simulink model "derpage6"  (R2015b)
settings: Solver=FixedStepDiscrete  SolverMode=SingleTasking  StartTime=0.0  StopTime=(12+350)*8  RelTol=1e-3
undefined symbols (not defined in the file or in its folder): rcosine
libraries: dspsrcs4 x2, dspsigops x2, dspstat3 x1
settings Model: Creator=coltmt  LastModifiedBy=coltmt

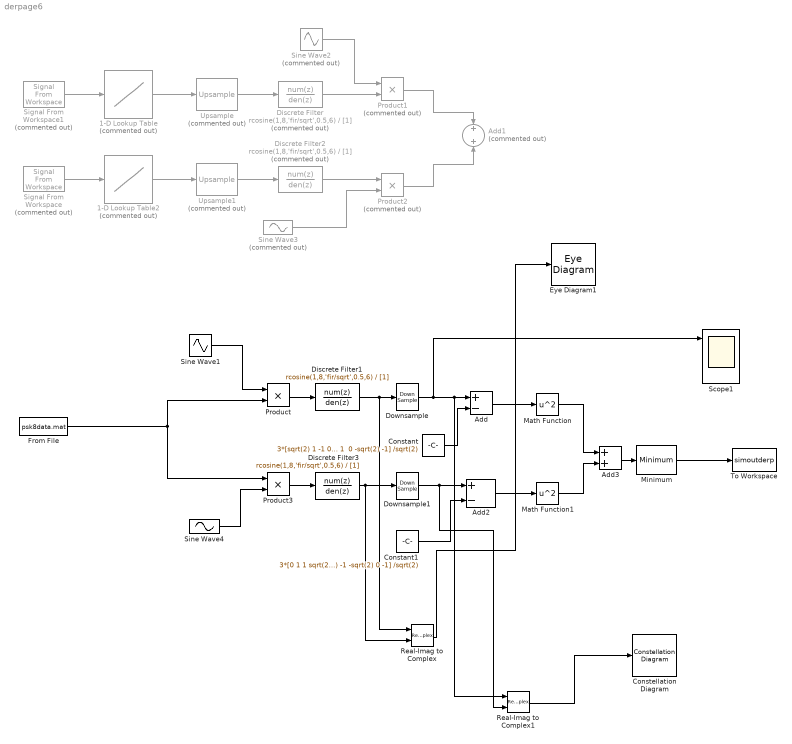
== system derpage6 ==
  1-D Lookup Table : Lookup_n-D  Commented=on  NumberOfTableDimensions=1  BreakpointsForDimension1=[0 1 2 3]  Table=[1 -1 1 -1]*3/sqrt(2)  InternalRulePriority=Speed  RndMeth=Simplest  InputSameDT=on
  1-D Lookup Table2 : Lookup_n-D  Commented=on  NumberOfTableDimensions=1  BreakpointsForDimension1=[0 1 2 3]  Table=[1 1 -1 -1]*3/sqrt(2)  InternalRulePriority=Speed  RndMeth=Simplest  InputSameDT=on
  Add : Sum  Inputs=+-
  Add1 : Sum  Commented=on
  Add2 : Sum  Inputs=+-
  Add3 : Sum
  Constant : Constant  Value="3*[sqrt(2) 1 -1 0 1  0 -sqrt(2) -1] /sqrt(2)"
  Constant1 : Constant  Value=3*[0 1 1 sqrt(2) -1 -sqrt(2) 0 -1] /sqrt(2)
  Constellation Diagram : ConstellationDiagram
  Discrete Filter : DiscreteFilter  Commented=on  Numerator=rcosine(1,8,'fir/sqrt',0.5,6)  Denominator=[1]
  Discrete Filter1 : DiscreteFilter  Numerator=rcosine(1,8,'fir/sqrt',0.5,6)  Denominator=[1]
  Discrete Filter2 : DiscreteFilter  Commented=on  Numerator=rcosine(1,8,'fir/sqrt',0.5,6)  Denominator=[1]
  Discrete Filter3 : DiscreteFilter  Numerator=rcosine(1,8,'fir/sqrt',0.5,6)  Denominator=[1]
  Downsample : DownSample  N=8  InputProcessing=Inherited (this choice will be removed - see release notes)  RateOptions=Allow multirate processing
  Downsample1 : DownSample  N=8  InputProcessing=Inherited (this choice will be removed - see release notes)  RateOptions=Allow multirate processing
  Eye Diagram1 : EyeDiagram
  From File : FromFile  FileName=psk8data.mat  SampleTime=1
  Math Function : Math  Operator=square  SaturateOnIntegerOverflow=on
  Math Function1 : Math  Operator=square  SaturateOnIntegerOverflow=on
  Minimum : dspstat3/Minimum  fcn=Index  reset=None  InputProcessing=Columns as channels (frame based)  indexBase=Zero  operateOver=Each column  Dimension=1  operation=minimum  roiEnable=off  roiType=Rectangles  roiPortion=Entire ROI  roiOutput=Individual statistics for each ROI  roiFlag=off  roundingMode=Floor  overflowMode=off
  Product : Product
  Product1 : Product  Commented=on
  Product2 : Product  Commented=on
  Product3 : Product
  Real-Imag to Complex : RealImagToComplex
  Real-Imag to Complex1 : RealImagToComplex
  Scope1 : Scope  NumInputPorts=3
  Signal From Workspace : dspsrcs4/Signal From Workspace  Commented=on  X=[0 2 1 3]  Ts=8  nsamps=1  OutputAfterFinalValue=Setting to zero  ignoreOrWarnInputAndFrameLengths=off  OutputFrames=off
  Signal From Workspace1 : dspsrcs4/Signal From Workspace  Commented=on  X=[0 2 1 3]  Ts=8  nsamps=1  OutputAfterFinalValue=Setting to zero  ignoreOrWarnInputAndFrameLengths=off  OutputFrames=off
  Sine Wave1 : Sin  Amplitude=sqrt(2)  Frequency=2*pi/4  Phase=pi/2  SampleTime=1
  Sine Wave2 : Sin  Commented=on  Amplitude=sqrt(2)  Frequency=2*pi/4  Phase=pi/2  SampleTime=1
  Sine Wave3 : Sin  Commented=on  Amplitude=-sqrt(2)  Frequency=2*pi/4  SampleTime=1
  Sine Wave4 : Sin  Amplitude=-sqrt(2)  Frequency=2*pi/4  SampleTime=1
  To Workspace : ToWorkspace  VariableName=simoutderp  SampleTime=-1
      settings: Save2DSignal=2-D array (concatenate along first dimension)
  Upsample : dspsigops/Upsample  Commented=on  N=8  phase=0  InputProcessing=Inherited (this choice will be removed - see release notes)  RateOptions=Allow multirate processing  ic=0  mode=Unused parameter value
  Upsample1 : dspsigops/Upsample  Commented=on  N=8  phase=0  InputProcessing=Inherited (this choice will be removed - see release notes)  RateOptions=Allow multirate processing  ic=0  mode=Unused parameter value
  wires:
  Signal From Workspace1/1 -> 1-D Lookup Table/1
  Signal From Workspace/1 -> 1-D Lookup Table2/1
  1-D Lookup Table/1 -> Upsample/1
  1-D Lookup Table2/1 -> Upsample1/1
  Upsample/1 -> Discrete Filter/1
  Upsample1/1 -> Discrete Filter2/1
  Discrete Filter/1 -> Product1/2
  Sine Wave2/1 -> Product1/1
  Discrete Filter2/1 -> Product2/1
  Sine Wave3/1 -> Product2/2
  Product2/1 -> Add1/2
  Product1/1 -> Add1/1
  Sine Wave1/1 -> Product/1
  Sine Wave4/1 -> Product3/2
  Product/1 -> Discrete Filter1/1
  Product3/1 -> Discrete Filter3/1
  Discrete Filter1/1 -> Real-Imag to Complex/1, Downsample/1
  Discrete Filter3/1 -> Real-Imag to Complex/2, Downsample1/1
  Downsample1/1 -> Real-Imag to Complex1/2, Add2/1
  Constant1/1 -> Add2/2
  Constant/1 -> Add/2
  Add/1 -> Math Function/1
  Add2/1 -> Math Function1/1
  Math Function/1 -> Add3/1
  Math Function1/1 -> Add3/2
  Add3/1 -> Minimum/1
  Minimum/1 -> To Workspace/1
  Downsample/1 -> Real-Imag to Complex1/1, Add/1, Scope1/1
  From File/1 -> Product/2, Product3/1
  Real-Imag to Complex/1 -> Eye Diagram1/1
  Real-Imag to Complex1/1 -> Constellation Diagram/1
